simulink library "vrlib"  (Simulink 7.5)
settings: Solver=ode45  SolverMode=SingleTasking  StartTime=0.0  StopTime=10.0  RelTol=1e-3
undefined symbols (not defined in the file or in its folder): gcbh, vrmfunc
libraries: vrlib x6, simulink x2
settings Model: ForwardingTableString=||__slOldName__||vrlib/Magellan Space Mouse||__slNewName__||vrlib/Space Mouse Input  Creator=Dluhos  LastModifiedBy=Houska  CovMetricSettings=d  ExtModeAutoUpdateStatusClock=off

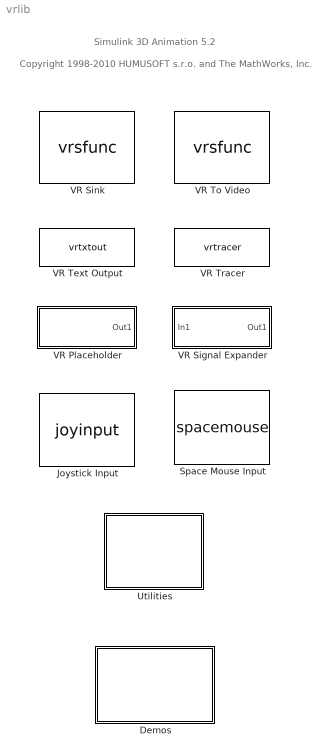
== system vrlib ==
  note: Copyright 1998-2010 HUMUSOFT s.r.o. and The MathWorks, Inc.
  note: Simulink 3D Animation 5.2
  Demos : Subsystem
      settings: OpenFcn=vrdemos
      mask Type: Simulink 3D Animation Demos
      mask Description: Double-click to open Simulink 3D Animation demos.
      mask Display: disp('Double-click to open\nSimulink 3D\nAnimation demos.')
  Joystick Input : S-Function  FunctionName=joyinput  Parameters=joyid, adjustports, forcefeed  EnableBusSupport=off  mask(Joystick Input){joyid=1, adjustports=off, forcefeed=off}
      mask prompts: joyid "Joystick ID:"; adjustports "Adjust I/O ports according to joystick capabilities"; forcefeed "Enable force-feedback input"
      mask help: Joystick input device driver.
      mask init:
      | label = 'image(imread(''joystickicon.png'')); port_label(''output'', 1, ''Axes''); port_label(''output'', 2, ''Buttons''); ';
      | porthandles = get_param(gcbh, 'PortHandles');
      | if numel(porthandles.Outport)>2
      |   label = [label 'port_label(''output'', 3, ''Point of View''); '];
      | end
      | if numel(porthandles.Inport)>0  label = [label 'port_label(''input'', 1, ''Force''); '];
      | end
      | set_param(gcbh, 'MaskDisplay', label);
      settings: CopyFcn=if ~vrmfunc('islibrary',gcbh) set_param(gcbh,'adjustports','on'); end
      mask Help: helpview(vrmfunc('FnHelpTopic'), 'vr_joystickinput');
      mask Display: image(imread('joystickicon.png')); port_label('output', 1, 'Axes'); port_label('output', 2, 'Buttons');
  Space Mouse Input : S-Function  FunctionName=spacemouse  Parameters=Port, OutputType, InitialPosition, InitialRotation, PositionSensitivity, RotationSensitivity, Dominant, NormalizeAngle, DisableTranslation, DisableRotation, PositionLow, PositionUp, EnableLimit  EnableBusSupport=off  mask(Space Mouse Input){Port=USB1, OutputType=Speed, Dominant=off, DisableTranslation=off, DisableRotation=off, NormalizeAngle=off, EnableLimit=off, PositionSensitivity=0.0001, RotationSensitivity=0.00001, InitialPosition=[0 0 0], InitialRotation=[0 0 0], PositionLow=[-100 -100 -100], PositionUp=[100 100 100]}
      mask prompts: OutputType "Output type:"; Dominant "Dominant mode"; DisableTranslation "Disable position movement"; DisableRotation "Disable rotation movement"; NormalizeAngle "Normalize output angle"; EnableLimit "Limit position"; PositionSensitivity "Position sensitivity:"; RotationSensitivity "Rotation sensitivity:"; InitialPosition "Initial position:"; InitialRotation "Initial rotation:"; PositionLow "Lower position limit:"; PositionUp "Upper position limit:"
      mask help: Space Mouse input device driver.
      mask Help: helpview(vrmfunc('FnHelpTopic'), 'vr_magellanspacemouse');
      mask StyleString: popup(COM1|COM2|COM3|COM4|USB1|USB2|USB3|USB4|USB),popup(Speed|Position|Viewpoint coordinates),checkbox,checkbox,checkbox,checkbox,checkbox,edit,edit,edit,edit,edit,edit
      mask CallbackString: spacemousemask|spacemousemask|||||spacemousemask||||||
      mask Display:
      | image(imread('spacemouseicon.png'))
      | port_label('output', 1, 'Translation')
      | port_label('output', 2, 'Rotation')
      | port_label('output', 3, 'Buttons')
  Utilities : Subsystem
      mask Display: image(imread('vrspanner.png'));
  VR Placeholder : Subsystem  mask(VR Placeholder){outwidth=1}
      mask prompts: outwidth "Output width"
      mask help: Generate a vector of VR Placeholder signals used for masking the unused or unaffected components of VRML fields.
      mask Help: helpview(vrmfunc('FnHelpTopic'), 'vr_vrplaceholder');
      mask Display:
      | text(0.1,0.5,'VR');
      | plot([0.4 0.4], [0.3 0.7]);
      | plot([0.4 0.9], [0.45 0.44]);
      | plot([0.4 0.9], [0.5 0.5]);
      | plot([0.4 0.9], [0.55 0.55]);
  VR Signal Expander : Subsystem  mask(VR Signal Expander){outwidth=4, outidx=[2 4]}
      mask prompts: outwidth "Output width"; outidx "Output signal indices"
      mask help:
      | Expand input vector into a fully qualified VRML field signal, filling the blank positions in the output port with the VR Placeholder signal.
      |
      | Input: The vector of inputs to be mapped into the output port.
      | Output width: The width of the output port.
      | Output signal indices: Positions of output vector at which the input signal elements appear. The remaining positions are filled with the VR Placeholder signal.
      mask init:
      | sel=ones(1,outwidth);
      | sel(outidx)=2:(length(outidx)+1);
      mask Help: helpview(vrmfunc('FnHelpTopic'), 'vr_vrsignalexpander');
      mask Display:
      | text(0.13,0.2,'VR');
      | plot([0.1 0.9],[0.6 0.9]);
      | plot([0.1 0.9],[0.55 0.8]);
      | plot([0.1 0.9],[0.5 0.5]);
      | plot([0.1 0.9],[0.45 0.2]);
      | plot([0.1 0.9],[0.4 0.1]);
  VR Sink : S-Function  InstantiateOnLoad=on  LoadFcn=vrmfunc('FnLoad', gcbh);  InitFcn=vrmfunc('FnInit', gcbh);  StartFcn=vrmfunc('FnSimStatus', gcbh, 'running')  StopFcn=vrmfunc('FnStop', gcbh)  FunctionName=vrsfunc  Parameters=WorldFileName, {}, FieldsWritten, AutoView, RemoteView, RemoteChange, SampleTime, WorldDescription  EnableBusSupport=off  mask(Virtual Reality Sink){SampleTime=0.1, ViewEnable=on, RemoteChange=off, RemoteView=on, FieldsWritten=, WorldFileName=, WorldDescription=, AutoView=off, VideoDimensions=[], FigureProperties={}}
      mask prompts: SampleTime "Sample Time"; ViewEnable "View"; RemoteChange "Remote Change"; RemoteView "Remote View"; FieldsWritten "Fields Written"; WorldFileName "World File Name"; WorldDescription "World Description"; VideoDimensions "Video Dimensions"; FigureProperties "Figure Properties"
      mask help: Controls the selected fields of a virtual world according to given inputs.
      mask init:
      | set_param(gcbh, 'MaskDisplay', vrmfunc('FnIcon'));
      settings: CopyFcn=vrmfunc('FnCopy', gcbh);  DeleteFcn=vrmfunc('FnDelete', gcbh);  PreSaveFcn=vrmfunc('FnPreSave', gcbh);  PauseFcn=vrmfunc('FnSimStatus', gcbh, 'paused');  ContinueFcn=vrmfunc('FnSimStatus', gcbh, 'running');  DestroyFcn=vrmfunc('FnDestroy', gcbh);  OpenFcn=vrmfunc('FnOpen', gcbh);  CloseFcn=vrmfunc('FnClose', gcbh);
      mask Help: helpview(vrmfunc('FnHelpTopic'), 'vr_vrsink');
      mask Display: image(imread('vrblockicon.png'));
  VR Text Output : M-S-Function  StartFcn=vrmfunc('FnSimStatus', gcbh, 'running')  StopFcn=vrmfunc('FnStop', gcbh)  FunctionName=vrtxtout  Parameters=VrmlFile, TxtNode, FormatString, Ts, ForceViewerOpen  mask(VR Text Output){VrmlFile=, TxtNode=, FormatString=, Ts=-1, ForceViewerOpen=off}
      mask prompts: VrmlFile "Associated VRML file:"; TxtNode "Associated Text node:"; FormatString "Format string:"; Ts "Sample time (-1 for inherited):"; ForceViewerOpen "Ensure that a viewer window is open during simulation"
      mask help:
      | Format the input data under control of the specified format string and output resulting string to the selected Text node in the associated virtual world.
      |
      | For possible format string definitions and block output see documentation for sprintf().
      | Exceptions:
      |   - VR Text Output supports only the \n escape non-printing character
      |   - %s and %c conversion characters are not allowed in the format string
      |
      | Input: The vector of values to be used as sprintf() arguments.
      settings: CopyFcn=vrmfunc('FnCopy', gcbh);  DeleteFcn=vrmfunc('FnDelete', gcbh);  PauseFcn=vrmfunc('FnSimStatus', gcbh, 'paused');  ContinueFcn=vrmfunc('FnSimStatus', gcbh, 'running');  DestroyFcn=vrmfunc('FnDestroy', gcbh);
      mask Help: helpview(vrmfunc('FnHelpTopic'), 'vr_vrtextoutput');
      mask Display:
      | text(0.1, 0.2, 'VR');
      | text(0.65, 0.5, 'TXT');
      | plot([0.35 0.55 0.45 0.55 0.45], [0.5 0.5 0.6 0.5 0.4]);
  VR To Video : S-Function  InstantiateOnLoad=on  LoadFcn=vrmfunc('FnLoad', gcbh);  InitFcn=vrmfunc('FnInit', gcbh);  StartFcn=vrmfunc('FnSimStatus', gcbh, 'running')  StopFcn=vrmfunc('FnStop', gcbh)  FunctionName=vrsfunc  Parameters=WorldFileName, {}, FieldsWritten, AutoView, RemoteView, RemoteChange, SampleTime, WorldDescription  EnableBusSupport=off  mask(Virtual Reality Sink){SampleTime=0.1, ViewEnable=on, RemoteChange=off, RemoteView=on, FieldsWritten=, WorldFileName=, WorldDescription=, AutoView=off, VideoDimensions=[200 320], FigureProperties={}}
      mask prompts: SampleTime "Sample Time"; ViewEnable "View"; RemoteChange "Remote Change"; RemoteView "Remote View"; FieldsWritten "Fields Written"; WorldFileName "World File Name"; WorldDescription "World Description"; VideoDimensions "Video Dimensions"; FigureProperties "Figure Properties"
      mask help: Controls the selected fields of a virtual world according to given inputs.
      mask init:
      | set_param(gcbh, 'MaskDisplay', vrmfunc('FnIcon'));
      settings: CopyFcn=vrmfunc('FnCopy', gcbh);  DeleteFcn=vrmfunc('FnDelete', gcbh);  PreSaveFcn=vrmfunc('FnPreSave', gcbh);  PauseFcn=vrmfunc('FnSimStatus', gcbh, 'paused');  ContinueFcn=vrmfunc('FnSimStatus', gcbh, 'running');  DestroyFcn=vrmfunc('FnDestroy', gcbh);  OpenFcn=vrmfunc('FnOpen', gcbh);  CloseFcn=vrmfunc('FnClose', gcbh);
      mask Help: helpview(vrmfunc('FnHelpTopic'), 'vr_vrtovideo');
      mask Display: image(imread('vrblockicon.png'));
  VR Tracer : M-S-Function  StartFcn=vrmfunc('FnSimStatus', gcbh, 'running')  StopFcn=vrmfunc('FnStop', gcbh)  FunctionName=vrtracer  Parameters=VrmlFile, ParentNode, MarkerName, UseLines, UseTriads, MarkerScale, MarkerColorSelection, MarkerColor, rgbval, Ts, ForceViewerOpen  mask(VR Tracer){VrmlFile=, ParentNode=, MarkerName=Tetrahedron, UseLines=on, UseTriads=on, MarkerScale=[1 1 1], MarkerColorSelection=Block input, MarkerColor=red, rgbval=[1 0 0], Ts=0.5, ForceViewerOpen=off}
      mask prompts: VrmlFile "Associated VRML file:"; ParentNode "Parent node (leave empty for root):"; MarkerName "Marker shape:"; UseLines "Connect markers with line segments"; UseTriads "Place a triad at each marker position"; MarkerScale "Marker scale:"; MarkerColorSelection "Marker color selection:"; MarkerColor "Marker color:"; rgbval "Marker color  (RGB):"; Ts "Sample time (-1 for inherited):"; ForceViewerOpen "Ensure that a viewer window is open during simulation"
      mask help:
      | Trace the trajectory of an object in the associated virtual scene.
      |
      | Marker nodes are created in regular time steps as children of specified parent node, or at the top level of scene hierarchy. You can create three types of markers - predefined shape markers, line segments connecting object positions in every time step and axis-aligned triads useful for orienting the trajectory in the 3D space.
      |
      | Object position input must correspond to the placement of the object in the scene hierarchy. If the traced object resides as a child of some parent object, define the parent object DEF name in the Parent node field. If the traced object resides at the top of the scene hierarchy (its position is defined in global scene coordinates), leave this field empty.
      |
      | Input: First input vector determines the position of the marker, second input (if enabled) represents the marker color.
      mask init:
      | label = ['text(0.8,0.2,''VR'');'...
      |          'plot([0.45 0.55 0.65 0.75 0.85 0.95],[0.3 0.35 0.42 0.52 0.67 0.85]);'...
      |          'text(0.55,0.405,''o'');'...
      |          'text(0.7,0.52,''o'');'...
      |          'text(0.85,0.703,''o'');'...
      |          'port_label(''input'', 1, ''Position'');'];
      | if MarkerColorSelection<=1
      |  label = [label 'port_label(''input'', 2, ''Color'');'];    
      | end
      | set_param(gcbh, 'MaskDisplay', label);
      settings: CopyFcn=vrmfunc('FnCopy', gcbh);  DeleteFcn=vrmfunc('FnDelete', gcbh);  PauseFcn=vrmfunc('FnSimStatus', gcbh, 'paused');  ContinueFcn=vrmfunc('FnSimStatus', gcbh, 'running');  DestroyFcn=vrmfunc('FnDestroy', gcbh);
      mask Help: helpview(vrmfunc('FnHelpTopic'), 'vr_tracer');
      mask StyleString: edit,edit,popup(None|Tetrahedron|Pyramid|Box|Octahedron|Sphere),checkbox,checkbox,edit,popup(Block input|Selected from color list|Defined as RGB values),popup(yellow|magenta|cyan|red|green|blue|white|black),edit,edit,checkbox
      mask CallbackString: ||||||vrtracer('MarkerColorSelectionCallback', gcbh);||||
      mask Display: text(0.8,0.2,'VR');plot([0.45 0.55 0.65 0.75 0.85 0.95],[0.3 0.35 0.42 0.52 0.67 0.85]);text(0.55,0.405,'o');text(0.7,0.52,'o');text(0.85,0.703,'o');port_label('input', 1, 'Position');port_label('input', 2, 'Color');

== system vrlib/Demos ==
  Empty : Subsystem

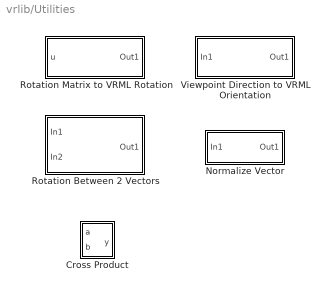
== system vrlib/Utilities ==
  Cross Product : Subsystem
      mask Type: Cross Product
      mask Description:
      | Cross product of two 3x1 vectors a=[a1 a2 a3], b=[b1 b2 b3].
      | y = a x b = (a2b3 - a3b2)i + (a3b1 - a1b3)j + (a1b2 - a2b1)k
      mask Help: helpview(vrmfunc('FnHelpTopic'), 'vr_crossproduct');
      mask Display:
      | plot([0.2 0.8],[0.8 0.2]);
      | plot([0.2 0.8],[0.2 0.8]);
  Normalize Vector : Subsystem  mask(Normalize Vector){maxzero=0}
      mask prompts: maxzero "Maximum modulus to treat vector as zero:"
      mask help:
      | Normalize a vector.
      | Output is the unit vector parallel to the input vector. Input can be vector of any size.
      | If the modulus of the input is lower or equal than specified, the output is set to zeros(size(u)).
      mask Help: helpview(vrmfunc('FnHelpTopic'), 'vr_normalizevector');
      mask Display: disp('Normalize')
  Rotation Between 2 Vectors : Subsystem
      mask Type: Rotation Between 2 Vectors
      mask Description:
      | Calculates a rotation between two vectors.
      | Output is a VRML rotation (specified as 4-element vector defining axis and angle ) needed to transform the first input to the second input. Both inputs must be 3x1 vectors.
      mask Help: helpview(vrmfunc('FnHelpTopic'), 'vr_rotbetween2vectors');
      mask Display:
      | text(0.1, 0.2, 'VR');
      | plot([0.47 0.54 0.6 0.68 0.62 0.68 0.65], [0.8 0.9 0.9 0.78 0.72 0.78 0.9]);
      | plot([0.3 0.7],[0.7 0.1]);
      | plot([0.55 0.8],[0.35 0.9]);
      | plot([0.55 0.4],[0.35 0.9]);
  Rotation Matrix to VRML Rotation : Subsystem  mask(Rotation Matrix to VRML Rotation){maxzero=1e-12}
      mask prompts: maxzero "Maximum value to treat input value as zero:"
      mask help:
      | Converts Rotation Matrix (defined columnwise as 3x3 matrix
      | or as 9-element column vector) into the Axis / Angle
      | rotation representation used for defining rotations in VRML.
      mask Help: helpview(vrmfunc('FnHelpTopic'), 'vr_rotmat2vrmlrot');
      mask Display:
      | text(0.1, 0.2, 'VR');
      | plot([0.2 0.4 0.4 0.2 0.2], [0.4 0.4 0.8 0.8 0.4]);
      | plot([0.25 0.25],[0.5 0.7]);
      | plot([0.3 0.3],[0.5 0.7]);
      | plot([0.35 0.35],[0.5 0.7]);
      | plot([0.47 0.65 0.55 0.65 0.55], [0.6 0.6 0.7 0.6 0.5]);
      | plot([0.85 0.80 0.77 0.75 0.73 0.73 0.75 0.80 0.85 0.90 0.92 0.95 0.95 0.95 0.91], [0.35 0.37 0.42 0.48 0.55 0.6 0.7 0.75 0.75 0.7 0.67 0.6 0.7 0.6 0.6]);
      | plot([0.75 0.9],[0.3 0.8]);
  Viewpoint Direction to VRML Orientation : Subsystem
      mask Type: Viewpoint Direction to VRML Orientation
      mask Description:
      | Converts viewpoint direction to VRML orientation.
      | Converts the viewpoint direction, specified by a vector of 3 elements, to a corresponding VRML viewpoint orientation (4-element VRML rotation vector).
      mask Help: helpview(vrmfunc('FnHelpTopic'), 'vr_vpdir2vrmlorient');
      mask Display:
      | text(0.1, 0.2, 'VR');
      | plot([0.25 0.4 0.35 0.4 0.4],[0.3 0.8 0.77 0.8 0.7]);
      | plot([0.45 0.65 0.55 0.65 0.55], [0.6 0.6 0.7 0.6 0.5]);
      | plot([0.85 0.80 0.77 0.75 0.73 0.73 0.75 0.80 0.85 0.90 0.92 0.95 0.95 0.95 0.91], [0.35 0.37 0.42 0.48 0.55 0.6 0.7 0.75 0.75 0.7 0.67 0.6 0.7 0.6 0.6]);
      | plot([0.75 0.9],[0.3 0.8]);

== system vrlib/VR Placeholder ==
  Constant : Constant  Value=NaN+zeros(1,outwidth)  OutDataType=sfix(16)  OutScaling=2^0
  Out1 : Outport  OutDataType=sfix(16)  OutScaling=2^0
  wires:
  Constant/1 -> Out1/1

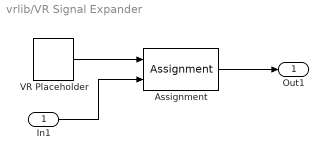
== system vrlib/VR Signal Expander ==
  In1 : Inport  OutDataType=sfix(16)  OutScaling=2^0
  Assignment : Assignment  IndexOptions=Index vector (dialog)  Indices=outidx  OutputSizes=[1 1]
  VR Placeholder : vrlib/VR Placeholder  outwidth=outwidth
  Out1 : Outport  OutDataType=sfix(16)  OutScaling=2^0
  wires:
  Assignment/1 -> Out1/1
  VR Placeholder/1 -> Assignment/1
  In1/1 -> Assignment/2

== system vrlib/Demos/Empty ==

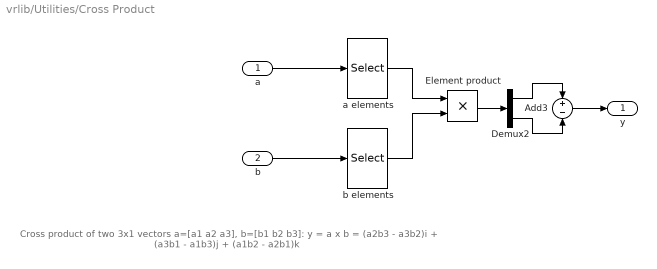
== system vrlib/Utilities/Cross Product ==
  note: Cross product of two 3x1 vectors a=[a1 a2 a3], b=[b1 b2 b3]:
      | y = a x b = (a2b3 - a3b2)i + (a3b1 - a1b3)j + (a1b2 - a2b1)k
  a : Inport  OutDataType=sfix(16)  OutScaling=2^0
  b : Inport  Port=2  OutDataType=sfix(16)  OutScaling=2^0
  Add3 : Sum  Inputs=+-  OutDataType=sfix(16)  OutScaling=2^-10
  Demux2 : Demux  Outputs=2
  Element product : Product  OutDataType=sfix(16)  OutScaling=2^0  RndMeth=Zero
  a elements : Selector  InputPortWidth=3  IndexOptions=Index vector (dialog)  Indices=[2 3 1 3 1 2]  OutputSizes=1
  b elements : Selector  InputPortWidth=3  IndexOptions=Index vector (dialog)  Indices=[3 1 2 2 3 1]  OutputSizes=1
  y : Outport  OutDataType=sfix(16)  OutScaling=2^0
  wires:
  Add3/1 -> y/1
  Demux2/2 -> Add3/2
  Demux2/1 -> Add3/1
  Element product/1 -> Demux2/1
  a/1 -> a elements/1
  b/1 -> b elements/1
  b elements/1 -> Element product/2
  a elements/1 -> Element product/1

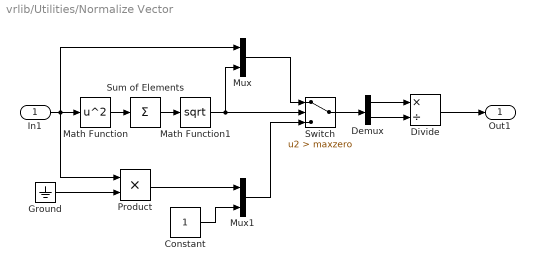
== system vrlib/Utilities/Normalize Vector ==
  In1 : Inport  OutDataType=sfix(16)  OutScaling=2^0
  Constant : Constant  OutDataType=sfix(16)  OutScaling=2^0
  Demux : Demux  Outputs=[-1 1]
  Divide : Product  Inputs=*/  OutDataType=sfix(16)  OutScaling=2^-10
  Ground : Ground
  Math Function : Math  Operator=square  OutDataType=sfix(16)  OutScaling=2^0  SaturateOnIntegerOverflow=on
  Math Function1 : Math  Operator=sqrt  OutDataType=sfix(16)  OutScaling=2^0  SaturateOnIntegerOverflow=on
  Mux : Mux  Inputs=2
  Mux1 : Mux  Inputs=2
  Product : Product  OutDataType=sfix(16)  OutScaling=2^0  RndMeth=Zero
  Sum of Elements : Sum  Inputs=+  OutDataType=sfix(16)  OutScaling=2^-10
  Switch : Switch  Criteria=u2 > Threshold  Threshold=maxzero  OutDataType=sfix(16)  OutScaling=2^0
  Out1 : Outport  OutDataType=sfix(16)  OutScaling=2^0
  wires:
  Ground/1 -> Product/2
  Product/1 -> Mux1/1
  Constant/1 -> Mux1/2
  Mux1/1 -> Switch/3
  Sum of Elements/1 -> Math Function1/1
  Math Function/1 -> Sum of Elements/1
  Demux/2 -> Divide/2
  Demux/1 -> Divide/1
  Switch/1 -> Demux/1
  Mux/1 -> Switch/1
  Math Function1/1 -> Mux/2, Switch/2
  In1/1 -> Product/1, Math Function/1, Mux/1
  Divide/1 -> Out1/1

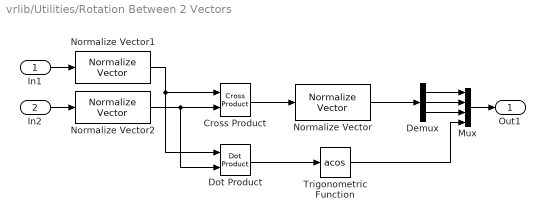
== system vrlib/Utilities/Rotation Between 2 Vectors ==
  In1 : Inport  OutDataType=sfix(16)  OutScaling=2^0
  In2 : Inport  Port=2  OutDataType=sfix(16)  OutScaling=2^0
  Cross Product : vrlib/Utilities/Cross Product
  Demux : Demux  Outputs=3
  Dot Product : simulink/Math Operations/Dot Product  InputSameDT=on  OutDataType=sfix(16)  OutScaling=2^-10  DoSatur=off
  Mux : Mux
  Normalize Vector : vrlib/Utilities/Normalize Vector  maxzero=0
  Normalize Vector1 : vrlib/Utilities/Normalize Vector  maxzero=0
  Normalize Vector2 : vrlib/Utilities/Normalize Vector  maxzero=0
  Trigonometric Function : Trigonometry  Operator=acos
  Out1 : Outport  OutDataType=sfix(16)  OutScaling=2^0
  wires:
  Dot Product/1 -> Trigonometric Function/1
  Demux/1 -> Mux/1
  Demux/2 -> Mux/2
  Demux/3 -> Mux/3
  Cross Product/1 -> Normalize Vector/1
  Trigonometric Function/1 -> Mux/4
  Normalize Vector/1 -> Demux/1
  Normalize Vector1/1 -> Dot Product/1, Cross Product/1
  Normalize Vector2/1 -> Dot Product/2, Cross Product/2
  In1/1 -> Normalize Vector1/1
  Mux/1 -> Out1/1
  In2/1 -> Normalize Vector2/1

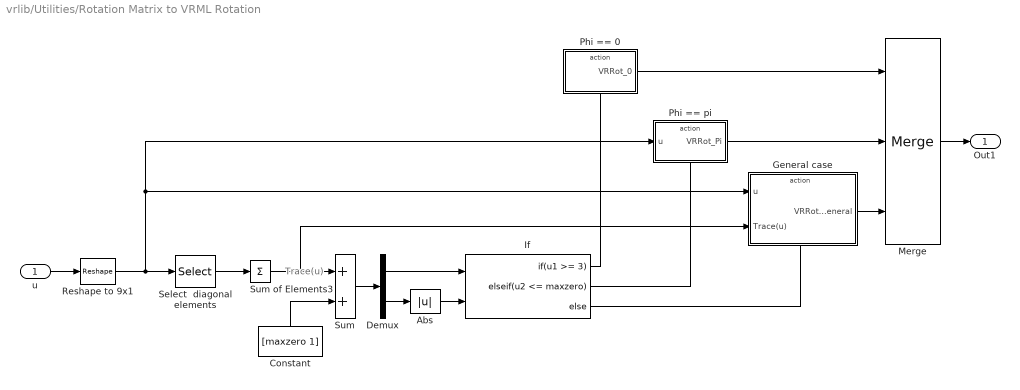
== system vrlib/Utilities/Rotation Matrix to VRML Rotation ==
  note: Trace(u)
  u : Inport  OutDataType=sfix(16)  OutScaling=2^0
  Abs : Abs  OutDataType=sfix(16)  OutScaling=2^0
  Constant : Constant  Value=[maxzero 1]  OutDataType=sfix(16)  OutScaling=2^0
  Demux : Demux  Outputs=2
  General case : Subsystem  TreatAsAtomicUnit=on
  If : If  NumInputs=2  IfExpression=u1 >= 3  ElseIfExpressions=u2 <= maxzero
  Merge : Merge  Inputs=3
  Phi == 0 : Subsystem  TreatAsAtomicUnit=on
  Phi == pi : Subsystem  TreatAsAtomicUnit=on
  Reshape to 9x1 : Reshape  OutputDimensions=[9,1]
  Select  diagonal elements : Selector  InputPortWidth=9  IndexOptions=Index vector (dialog)  Indices=[1 5 9]  OutputSizes=1
  Sum : Sum  OutDataType=sfix(16)  OutScaling=2^0
  Sum of Elements3 : Sum  Inputs=+  OutDataType=sfix(16)  OutScaling=2^-10
  Out1 : Outport  OutDataType=sfix(16)  OutScaling=2^0
  wires:
  Demux/1 -> If/1
  Demux/2 -> Abs/1
  Sum/1 -> Demux/1
  Abs/1 -> If/2
  Sum of Elements3/1 -> Sum/1, General case/2(Trace(u))
  u/1 -> Reshape to 9x1/1
  If/1 -> Phi == 0/Action
  Phi == 0/1(VRRot_0) -> Merge/1
  If/2 -> Phi == pi/Action
  If/3 -> General case/Action
  Phi == pi/1(VRRot_Pi) -> Merge/2
  General case/1(VRRot_General) -> Merge/3
  Merge/1 -> Out1/1
  Constant/1 -> Sum/2
  Reshape to 9x1/1 -> General case/1(u), Phi == pi/1(u), Select  diagonal elements/1
  Select  diagonal elements/1 -> Sum of Elements3/1

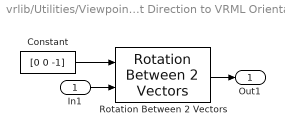
== system vrlib/Utilities/Viewpoint Direction to VRML Orientation ==
  In1 : Inport  OutDataType=sfix(16)  OutScaling=2^0
  Constant : Constant  Value=[0 0 -1]  OutDataType=sfix(16)  OutScaling=2^0
  Rotation Between 2 Vectors : vrlib/Utilities/Rotation Between 2 Vectors
  Out1 : Outport  OutDataType=sfix(16)  OutScaling=2^0
  wires:
  Constant/1 -> Rotation Between 2 Vectors/1
  Rotation Between 2 Vectors/1 -> Out1/1
  In1/1 -> Rotation Between 2 Vectors/2

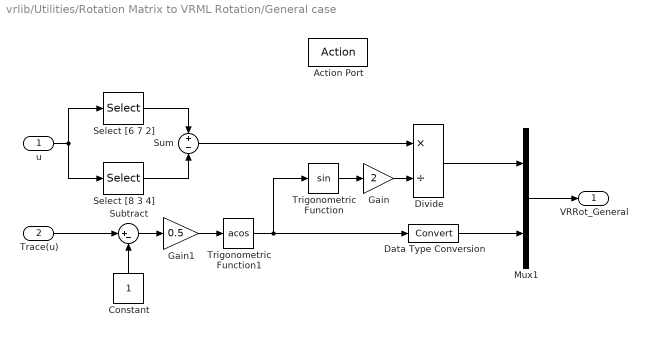
== system vrlib/Utilities/Rotation Matrix to VRML Rotation/General case ==
  u : Inport  OutDataType=sfix(16)  OutScaling=2^0
  Trace(u) : Inport  Port=2  OutDataType=sfix(16)  OutScaling=2^0
  Action Port : ActionPort  PropagateVarSize=During execution
  Constant : Constant  OutDataType=sfix(16)  OutScaling=2^0
  Data Type Conversion : DataTypeConversion  OutDataType=sfix(16)  OutScaling=2^0
  Divide : Product  Inputs=*/  OutDataType=sfix(16)  OutScaling=2^-10
  Gain : Gain  Gain=2  ParameterDataType=sfix(16)  ParameterScaling=2^0  OutDataType=sfix(16)  OutScaling=2^0
  Gain1 : Gain  Gain=0.5  ParameterDataType=sfix(16)  ParameterScaling=2^0  OutDataType=sfix(16)  OutScaling=2^0
  Mux1 : Mux  Inputs=2
  Select [6 7 2] : Selector  InputPortWidth=9  IndexOptions=Index vector (dialog)  Indices=[6 7 2]  OutputSizes=1
  Select [8 3 4] : Selector  InputPortWidth=9  IndexOptions=Index vector (dialog)  Indices=[8 3 4]  OutputSizes=1
  Subtract : Sum  Inputs=|+-  OutDataType=sfix(16)  OutScaling=2^-10
  Sum : Sum  Inputs=+-  OutDataType=sfix(16)  OutScaling=2^0
  Trigonometric Function : Trigonometry
  Trigonometric Function1 : Trigonometry  Operator=acos
  VRRot_General : Outport  OutDataType=sfix(16)  OutScaling=2^0
  wires:
  Data Type Conversion/1 -> Mux1/2
  Trigonometric Function/1 -> Gain/1
  Gain/1 -> Divide/2
  Mux1/1 -> VRRot_General/1
  Divide/1 -> Mux1/1
  Trace(u)/1 -> Subtract/1
  Constant/1 -> Subtract/2
  Subtract/1 -> Gain1/1
  Gain1/1 -> Trigonometric Function1/1
  Trigonometric Function1/1 -> Trigonometric Function/1, Data Type Conversion/1
  u/1 -> Select [6 7 2]/1, Select [8 3 4]/1
  Sum/1 -> Divide/1
  Select [6 7 2]/1 -> Sum/1
  Select [8 3 4]/1 -> Sum/2

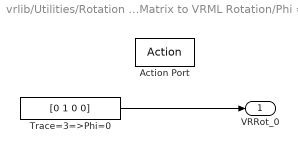
== system vrlib/Utilities/Rotation Matrix to VRML Rotation/Phi == 0 ==
  Action Port : ActionPort  PropagateVarSize=During execution
  Trace=3=>Phi=0 : Constant  Value=[0 1 0 0]  OutDataType=sfix(16)  OutScaling=2^0  SampleTime=Inf
  VRRot_0 : Outport  OutDataType=sfix(16)  OutScaling=2^0  InitialOutput=[0 1 0 0]
  wires:
  Trace=3=>Phi=0/1 -> VRRot_0/1

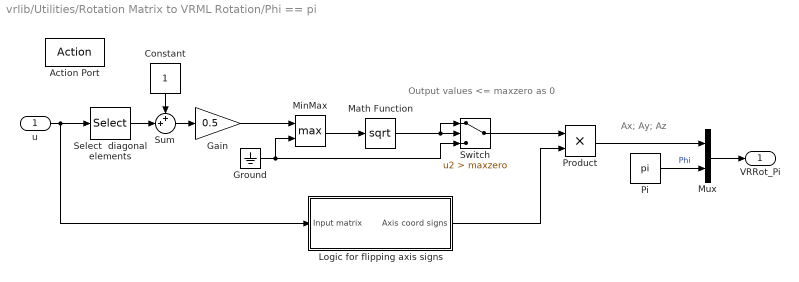
== system vrlib/Utilities/Rotation Matrix to VRML Rotation/Phi == pi ==
  note: Ax; Ay; Az
  note: Output values <= maxzero as 0
  u : Inport  OutDataType=sfix(16)  OutScaling=2^0
  Action Port : ActionPort  PropagateVarSize=During execution
  Constant : Constant  OutDataType=sfix(16)  OutScaling=2^0
  Gain : Gain  Gain=0.5  ParameterDataType=sfix(16)  ParameterScaling=2^0  OutDataType=sfix(16)  OutScaling=2^0
  Ground : Ground
  Logic for flipping axis signs : Subsystem
  Math Function : Math  Operator=sqrt  OutputSignalType=real  OutDataType=sfix(16)  OutScaling=2^0  SaturateOnIntegerOverflow=on
  MinMax : MinMax  Function=max  Inputs=2  OutDataType=sfix(16)  OutScaling=2^0
  Mux : Mux  Inputs=2
  Pi : Constant  Value=pi  OutDataType=sfix(16)  OutScaling=2^0  SampleTime=Inf
  Product : Product  OutDataType=sfix(16)  OutScaling=2^0  RndMeth=Zero
  Select  diagonal elements : Selector  InputPortWidth=9  IndexOptions=Index vector (dialog)  Indices=[1 5 9]  OutputSizes=1
  Sum : Sum  Inputs=++|  OutDataType=sfix(16)  OutScaling=2^0
  Switch : Switch  Criteria=u2 > Threshold  Threshold=maxzero  OutDataType=sfix(16)  OutScaling=2^0
  VRRot_Pi : Outport  OutDataType=sfix(16)  OutScaling=2^0  InitialOutput=[0 0 0 pi]
  wires:
  Pi/1 -> Mux/2  "Phi"
  Sum/1 -> Gain/1
  Select  diagonal elements/1 -> Sum/2
  Constant/1 -> Sum/1
  u/1 -> Select  diagonal elements/1, Logic for flipping axis signs/1(Input matrix)
  Mux/1 -> VRRot_Pi/1
  Ground/1 -> Switch/3, MinMax/2
  Gain/1 -> MinMax/1
  Product/1 -> Mux/1
  Logic for flipping axis signs/1(Axis coord signs) -> Product/2
  MinMax/1 -> Math Function/1
  Switch/1 -> Product/1
  Math Function/1 -> Switch/1, Switch/2

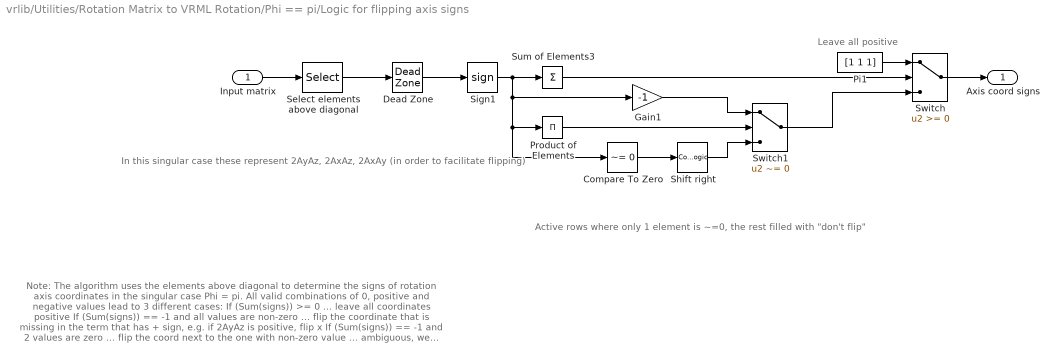
== system vrlib/Utilities/Rotation Matrix to VRML Rotation/Phi == pi/Logic for flipping axis signs ==
  note: Note:
      | The algorithm uses the elements above diagonal to determine the signs of rotation axis coordinates
      | in the singular case Phi = pi. All valid combinations of 0, positive and negative values lead to 3 different cases:
      | If (Sum(signs)) >= 0 ... leave all coordinates positive
      | If (Sum(signs)) == -1 and all values are non-zero ... flip the coordinate that is missing in the term that has + sign, e.g. if 2AyAz is positive, flip x
      | If (Sum(signs)) == -1 and 2 values are zero ... flip the coord next to the one with non-zero value ... ambiguous, we have chosen shift right
  note: In this singular case these
      | represent 2AyAz, 2AxAz, 2AxAy
      | (in order to facilitate flipping)
  note: Active rows where
      | only 1 element is ~=0,
      | the rest filled with
      | "don't flip"
  note: Leave all positive
  Input matrix : Inport  OutDataType=sfix(16)  OutScaling=2^0
  Compare To Zero : simulink/Logic and Bit Operations/Compare To Zero  SystemSampleTime=-1  relop=~=  LogicOutDataTypeMode=boolean  ZeroCross=off
  Dead Zone : DeadZone  LowerValue=-maxzero  UpperValue=maxzero  SaturateOnIntegerOverflow=on
  Gain1 : Gain  Gain=-1  ParameterDataType=sfix(16)  ParameterScaling=2^0  OutDataType=sfix(16)  OutScaling=2^0
  Pi1 : Constant  Value=[1 1 1]  OutDataType=sfix(16)  OutScaling=2^0  SampleTime=Inf
  Product of Elements : Product  Inputs=*  OutDataType=sfix(16)  OutScaling=2^-10
  Select elements above diagonal : Selector  InputPortWidth=9  IndexOptions=Index vector (dialog)  Indices=[8 7 4]  OutputSizes=1
  Shift right : CombinatorialLogic  TruthTable=[1 1 1;-1 1 1;1 1 -1;1 1 1;1 -1 1;1 1 1;1 1 1;1 1 1]
  Sign1 : Signum
  Sum of Elements3 : Sum  Inputs=+  OutDataType=sfix(16)  OutScaling=2^-10
  Switch : Switch  OutDataType=sfix(16)  OutScaling=2^0
  Switch1 : Switch  Criteria=u2 ~= 0  OutDataType=sfix(16)  OutScaling=2^0
  Axis coord signs : Outport  OutDataType=sfix(16)  OutScaling=2^0
  wires:
  Input matrix/1 -> Select elements above diagonal/1
  Select elements above diagonal/1 -> Dead Zone/1
  Dead Zone/1 -> Sign1/1
  Sign1/1 -> Sum of Elements3/1, Compare To Zero/1, Product of Elements/1, Gain1/1
  Sum of Elements3/1 -> Switch/2
  Product of Elements/1 -> Switch1/2
  Pi1/1 -> Switch/1
  Switch1/1 -> Switch/3
  Switch/1 -> Axis coord signs/1
  Gain1/1 -> Switch1/1
  Shift right/1 -> Switch1/3
  Compare To Zero/1 -> Shift right/1
